simulink model "VSM_specComp_DC_22a"  (R2022a)
settings: Solver=ode3  StartTime=0.0  StopTime=4  FixedStep=HWSampleTime  RelTol=1e-3
PostLoadFcn:
  | EXEC_MODE=ExecutionMode.SIMULATION;
  | %Sim_TP33_VSM_HSS_init
InitFcn:
  | %EXEC_MODE=ExecutionMode.SIMULATION;
  | %Sim_TP33_VSM_HSS_init
StopFcn:
  | %sim2struct
undefined symbols (not defined in the file): ControlSampleTime, DiscIntNeverNeededParam, fault_dur, Grid, HWSampleTime, Ion, LCL, Lithium, Manage, Param, SM, t_fault, V_DC, VSMCTRL
libraries: FriedrichLibrary x76, simulink x32, TriphaseHardwaremodule x24, spsThreePhaseSeriesRLCBranchLib x8, spsThreePhaseVIMeasurementLib x8, spsThreePhaseBreakerLib x8, spsGroundLib x4, spsUniversalBridgeLib x4, spsVoltageMeasurementLib x4, spsEdgeDetectorLib x4, spsMeanLib x4, simulink_extras x4
(part 10 of 10)

== matlab function VSM_specComp_DC_22a/VSM_1/VSM1/VSM/MANAGEMENT/Subsystem1/Subsystem/MATLAB Function1 ==
  data: i_inv input; i_sp output; PQ_out input; CC output; i_abs input; der input; set1 output; U_cap input; i_pq_pre input; i_abs_pre input; u_diff input
function [i_sp, CC, set1]= fcn(i_inv, PQ_out, i_abs, der, U_cap, i_pq_pre, i_abs_pre, u_diff)
    persistent set
    if isempty(set)
        set = 0;
    end

    persistent d
    if isempty(d)
        d = 0;
    end    
    
    persistent x
    if isempty(x)
        x = 0;
    end    
    
    persistent i_sp_old
    if isempty(i_sp_old)
        i_sp_old = [0 0];
    end
    
    persistent a
    if isempty(a)
        a = [10 10 10 10];
    end
    
    persistent a_u
    if isempty(a_u)
        a_u = [10 10 10 10 10 10 10 10 10 10 10 10];
    end
    
    persistent zero
    if isempty(zero)
        zero = [10 10 10 10];
    end  
    
    persistent time
      if isempty(time)
        time = 0;
      end    
    time = time +1;
    
    persistent regler
    if isempty(regler)
        regler = 0;
    end    
    persistent sdf
    if isempty(sdf)
        sdf = 1;
    end  

    CC = false;
    i_sp = [0 0];
    f = 0;
    adf = 10;
    %i_abs = sqrt(i_inv(1)^2 + i_inv(2)^2 + i_inv(3)^2);
    
    if i_abs >= 1.05 && d == 0 % && U_cap <= 0.9 %momentan hohe Spannung
        CC = true;
        set = 1;
    end
    
    if set == 1
        
      i_sp = [0 0];
   CC = true;
    end
    
    if i_abs <= 1 && set == 1 %&& sum(a>1) <= 1
        
        set = 2;
        
        i_sp_old = [i_inv(1) i_inv(2)];
       CC = true;

    end
    a = [a(2:4) i_abs];
    a_u = [a_u(2:12) PQ_out(2)/U_cap];
    
    if set == 2 %&& sum(a>1) <= 1 %&& sum(a_u>0.4) == 0
        [angle, mag] = cart2pol(i_sp_old(1), i_sp_old(2));
        d = 2;
        if PQ_out(2)/U_cap <=0
            f = 6;
        else
        f = 6*(1 - PQ_out(2)/U_cap);            %%lieber PI benutzen und/oder Faktoren in Abhängigkeit von dU machen
        %f = ( PQ_out(2)/U_cap/0.5)^0.5;
        end
        regler = regler - +0.1/2/1.1*(1 - PQ_out(2)/U_cap)+angle*sdf;
i_sp = [regler, 1];
sdf=0;
     %   regler = regler + 0.98 - PQ_out(2)/U_cap;
%f = regler*0.1;
%         if abs(0-U_der1)<= 0.5
%             zero = [zero(2:4) 0]
%         else
%             zero = [zero(2:4) 10]
%         end
%         
%         if sum(zero) == 0 && U_der2 <0
%             f = 0;
%         end
        
        %i_sp = [angle-1/100*f, 1];
        
        [i_sp(1), i_sp(2)]  = pol2cart(i_sp(1), i_sp(2));
        
%         if sum(zero) == 0 && U_der2 <0
%             set = 3;
%             i_sp = [i_inv(1) i_inv(2)];
%         end
        i_sp_old = i_sp;
        CC = true;
        
%         if U_der2 <= 0 && abs(0-U_der1)<= 0.5
%             
%             f = 0;
%         end
%         


    end
    
%     letzte Bedingung ist ungünstig. Entweder Erfüllung des
%     Stromsollwertes mit i_sp~=0, oder Counter in set 2
    
%     if abs(PQ_out(1)) <= 0.05 && PQ_out(2) > 0 && set == 2 && sqrt(PQ_out(1)^2 + PQ_out(2)^2) > 0.1
%               
%        set = 3
%        
%        %i_sp_old = [i_inv(1) i_inv(2)];          % nimmt den aktuellen Stromwert für Blindstrombestimmung
%         CC = true;
%     end    

    if set == 2 && abs(der) <= 5 % PQ_out(2)/U_cap >= 0.99 &&PQ_out(2)/U_cap <= 1.01 && %&& sum(a_u>0.95) == 12 
        %set = 3;
        CC = true;
        adf = 20;
        set = 4;
        CC = false;
        x = 0;
       %i_sp_old = [0 0];
       i_sp_old = [i_inv(1) i_inv(2)];
   %set = 3;
    end

    if set == 3
       
     % i_sp = i_sp_old * (1 - U_cap);
      i_sp = i_sp_old * 1;
      %i_sp = [0.28 -1.06];
       CC = true;
x = x +1;

    if x >= 25*4
        set = 4;
        CC = false;
        x = 0;
        i_sp_old = [0 0];
    end
    end
    
   if 0.115 == time/8000 
        set = 4;
        CC = false;
        x = 0;
        i_sp_old = [0 0];
   end
    
      if set == 4
        set = 4;
        CC = false;
        x = 0;
        i_sp_old = [0 0];
    end
%     
%     % Regelabweichung nicht sonderlich relevant-> lässt CC nur länger
%     % ausgelöst
%     
%     if set == 3 && abs(der(1)) <= 5 && abs(der(2)) <= 5 && abs(i_inv(1)-i_sp(1)) <= 0.05 && abs(i_inv(2)-i_sp(2)) <= 0.05
%         CC = false;
%         set = 0;
%         i_sp_old = [0 0];
%     end
%     

   
    
    %% Spannungswiederkehr ohne Überstrom
    
%     if U_cap >= 0.9
%         CC = true;
%         set = 5;
%         x= x +1;
%     end
%     
%     if x >= 2
%         CC = false;
%         set = 0;
%         x = 0;
%     end
%     %% Spannungswiederkehr
%     
    if i_abs >= 1.05 && U_cap >= 0.6 && set == 4
        CC = true;
        set = 5;
    end
    
    if u_diff >= 0.1 && set ==4 && U_cap >= 0.9
        set = 5;
    end
    
    if set == 5
        
      i_sp = [0 0];
   CC = true;
    end

    if i_abs <= 1 && set == 5 %&&i_abs <= i_abs_pre
        
        set = 6;
        
        i_sp_old = [i_inv(1) i_inv(2)];
       CC = true;

    end
    q=0;
    f=0;
%     if set == 6  %% für gleiches P und Q bei gleicher Stromzeigerlänge
%         [angle, mag] = cart2pol(i_sp_old(1), i_sp_old(2));
%         
%         f = 6*(PQ_pre(1) - PQ_out(1));            %%lieber PI benutzen und/oder Faktoren in Abhängigkeit von dU machen
%         q = 6*(PQ_pre(2) - PQ_out(2));
%         i_sp = [angle-1/100*f-1/100*q, 0.92];
%         
%         [i_sp(1), i_sp(2)]  = pol2cart(i_sp(1), i_sp(2));
%         
%         i_sp_old = i_sp;
%         CC = true;     
%     end
        if set == 6  %% für gleichen Wirkstrom und Blindstrom
        [angle, mag] = cart2pol(i_sp_old(1), i_sp_old(2));
        q = 2/2*2*(i_pq_pre(2) - PQ_out(2)/U_cap);          %sorgt dafür, dass in den richtigen Quadranten gezogen wird
        f = 1/2*2*(i_pq_pre(1) - PQ_out(1)/U_cap);           
        i_sp = [angle-1/100*f-1/100*q, i_abs_pre];
        
        [i_sp(1), i_sp(2)]  = pol2cart(i_sp(1), i_sp(2));
        
        i_sp_old = i_sp;
        CC = true;     
    end

    if PQ_out(1)/U_cap >= i_pq_pre(1)-0.01 &&PQ_out(1)/U_cap <= i_pq_pre(1)+0.01 && set == 6 && abs(der) <= 2%time/8000 >= 0.23
                CC = false;
        set = 0;
        i_sp_old = [0 0];
    end
        
% %     letzte Bedingung ist ungünstig. Entweder Erfüllung des
% %     Stromsollwertes mit i_sp~=0, oder Counter in set 2
%     
%     if abs(PQ_out(2)) <= 0.05 && PQ_out(1) > 0 && set == 6 && sqrt(PQ_out(1)^2 + PQ_out(2)^2) > 0.1
%               
%        set = 7
%         CC = true;
%     end    
%    
%     if set == 7
%        
%       i_sp = i_sp_old;
%        CC = true;
%     end
%     
%     % Regelabweichung nicht sonderlich relevant-> lässt CC nur länger
%     % ausgelöst
%     
%     if set == 7 && abs(der(1)) <= 10 && abs(der(2)) <= 10 && abs(i_inv(1)-i_sp(1)) <= 0.05 && abs(i_inv(2)-i_sp(2)) <= 0.05
%         CC = false;
%         set = 0;
%         i_sp_old = [0 0];
%     end
    [angle, mag] = cart2pol(i_sp_old(1), i_sp_old(2));
     set1 = angle;%regler; %angle;
